simulink model "doublemass"  (R2018a)
settings: Solver=FixedStepAuto  StartTime=0.0  StopTime=10.0  FixedStep=0.02  RelTol=1e-3
values from neighbouring files (symbols this model uses):
  a_max = [10,]    [doublemass_para.m]
  a_min = [-10,]    [doublemass_para.m]
  adva_max = [0.001,0.001,0.001,0.001,]    [doublemass_para.m]
  adva_min = [-0.001,-0.001,-0.001,-0.001,]    [doublemass_para.m]
  ka = 50    [doublemass_para.m]
  m1 = 10    [doublemass_para.m]
  m2 = 10    [doublemass_para.m]
  x_ini = [x1_o, x1dot_o, x2_o, x2dot_o,]    [doublemass_para.m]
  x_max = [9999, 9999, 9999, 9999,]    [doublemass_para.m]
  x_min = [-9999, -9999, -9999, -9999,]    [doublemass_para.m]
libraries: simulink x1
settings Model: TunableVars=a_max,a_min,adva_max,adva_min,x_ini,x_max,x_min  TunableVarsStorageClass=Auto,Auto,Auto,Auto,Auto,Auto,Auto  TunableVarsTypeQualifier=,,,,,,  OrderedModelArguments=off  Creator=hjzsj  LastModifiedBy=Jet
settings DataIOCC: ReturnWorkspaceOutputs=on
settings OptimizationCC: DefaultParameterBehavior=Inlined  UseDivisionForNetSlopeComputation=on  UseFloatMulNetSlope=on  PassReuseOutputArgsAs=Individual arguments  NoFixptDivByZeroProtection=on  EfficientFloat2IntCast=on  LifeSpan=1  OptimizeBlockOrder=speed  DifferentSizesBufferReuse=on
settings DebuggingCC: ParameterTunabilityLossMsg=error
settings HardwareCC: ProdLongLongMode=on
settings SFSimCC: SimUseLocalCustomCode=on  MATLABDynamicMemAlloc=off
settings RTWCC: SystemTargetFile=ert.tlc  GenCodeOnly=on  TemplateMakefile=ert_default_tmf  PostCodeGenCommand=mat2json  RTWUseLocalCustomCode=on  TargetLang=C++
settings CodeAppCC: ForceParamTrailComments=on  IgnoreCustomStorageClasses=off  OperatorAnnotations=on  SimulinkDataObjDesc=on  SFDataObjDesc=on  CustomSymbolStrGlobalVar=rt$N$M  CustomSymbolStrType=$N$M  CustomSymbolStrFcn=$N$M$F  CustomSymbolStrMacro=$N$M  InsertBlockDesc=on
settings ERTTargetCC: TargetLangStandard=C++03 (ISO)  GenerateSampleERTMain=on  CombineSignalStateStructs=on  MultiInstanceERTCode=on  CodeInterfacePackaging=C++ class  SupportComplex=off  SupportContinuousTime=on  InlinedParameterPlacement=NonHierarchical  RootIOFormat=Structure reference  ERTCustomFileTemplate=example_file_process.tlc  ERTFilePackagingFormat=CompactWithDataFile

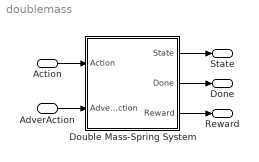
== system doublemass ==
  Action : Inport
  AdverAction : Inport  Port=2
  Double Mass-Spring System : Subsystem
  State : Outport  VectorParamsAs1DForOutWhenUnconnected=on
  Done : Outport  Port=2  VectorParamsAs1DForOutWhenUnconnected=on
  Reward : Outport  Port=3  VectorParamsAs1DForOutWhenUnconnected=on
  wires:
  Double Mass-Spring System/1(State) -> State/1
  Double Mass-Spring System/2(Done) -> Done/1
  Action/1 -> Double Mass-Spring System/1(Action)
  Double Mass-Spring System/3(Reward) -> Reward/1
  AdverAction/1 -> Double Mass-Spring System/2(AdverAction)

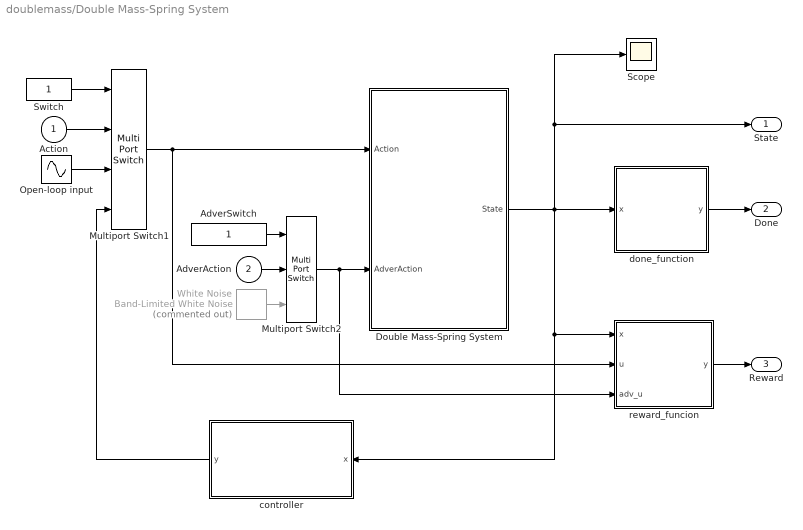
== system doublemass/Double Mass-Spring System ==
  Action : Inport
  AdverAction : Inport  Port=2
  AdverSwitch : Constant
  Double Mass-Spring System : Subsystem
  Multiport Switch1 : MultiPortSwitch
  Multiport Switch2 : MultiPortSwitch  Inputs=2
  Open-loop input : Sin  SampleTime=0
  Scope : Scope
  Switch : Constant
  White Noise : simulink/Sources/Band-Limited White Noise  Commented=on  Cov=[0.5]  Ts=0.02  seed=[23341]
  controller : MATLAB Function  TreatAsAtomicUnit=on
  done_function : MATLAB Function  TreatAsAtomicUnit=on
  reward_funcion : MATLAB Function  TreatAsAtomicUnit=on
  State : Outport  VectorParamsAs1DForOutWhenUnconnected=on
  Done : Outport  Port=2  VectorParamsAs1DForOutWhenUnconnected=on
  Reward : Outport  Port=3  VectorParamsAs1DForOutWhenUnconnected=on
  wires:
  done_function/1(y) -> Done/1
  reward_funcion/1(y) -> Reward/1
  controller/1(y) -> Multiport Switch1/4
  Switch/1 -> Multiport Switch1/1
  Action/1 -> Multiport Switch1/2
  Double Mass-Spring System/1(State) -> controller/1(x), reward_funcion/1(x), done_function/1(x), Scope/1, State/1
  Multiport Switch1/1 -> reward_funcion/2(u), Double Mass-Spring System/1(Action)
  Open-loop input/1 -> Multiport Switch1/3
  Multiport Switch2/1 -> reward_funcion/3(adv_u), Double Mass-Spring System/2(AdverAction)
  AdverSwitch/1 -> Multiport Switch2/1
  White Noise/1 -> Multiport Switch2/3
  AdverAction/1 -> Multiport Switch2/2

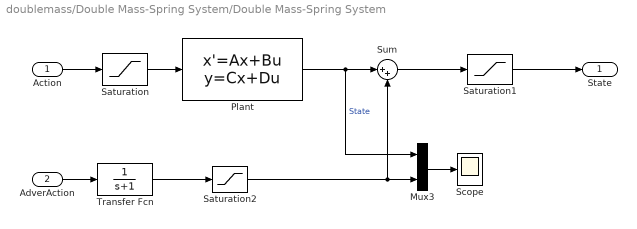
== system doublemass/Double Mass-Spring System/Double Mass-Spring System ==
  Action : Inport
  AdverAction : Inport  Port=2
  Mux3 : Mux  Inputs=2
  Plant : StateSpace  A=[0 1 0 0; -ka/m1 0 ka/m1 0; 0 0 0 1;ka/m2 0 -ka/m2 0]  B=[0; 1; 0; 0]  C=[1 0 0 0;0 1 0 0;0 0 1 0;0 0 0 1]  D=zeros(4,1)  InitialCondition=x_ini
  Saturation : Saturate  UpperLimit=a_max  LowerLimit=a_min
  Saturation1 : Saturate  UpperLimit=x_max  LowerLimit=x_min
  Saturation2 : Saturate  UpperLimit=adva_max  LowerLimit=adva_min
  Scope : Scope
  Sum : Sum  Inputs=|++
  Transfer Fcn : TransferFcn  Denominator=[1 1]
  State : Outport  VectorParamsAs1DForOutWhenUnconnected=on
  wires:
  Saturation/1 -> Plant/1
  Action/1 -> Saturation/1
  Saturation1/1 -> State/1
  Transfer Fcn/1 -> Saturation2/1
  Mux3/1 -> Scope/1
  AdverAction/1 -> Transfer Fcn/1
  Saturation2/1 -> Sum/2, Mux3/2
  Sum/1 -> Saturation1/1
  Plant/1 -> Mux3/1, Sum/1  "State"

== matlab function doublemass/Double Mass-Spring System/controller ==
  data: x input size=4; y output
function y = fcn(x)
done = (abs(x(1)) > 2.4)||(abs(x(3)) > 0.2094);
y = done;

== matlab function doublemass/Double Mass-Spring System/done_function ==
  data: x input; y output
function y = fcn(x)
done = (  (abs(x(3))>5) || ((abs(x(3)-0)<0.01) && (abs(x(4))<0.01)) || (x(3)>x(1))  );
y = done;

== matlab function doublemass/Double Mass-Spring System/reward_funcion ==
  data: x input; y output; u input; adv_u input
function y = fcn(x, u, adv_u)
reward = -(x(3)-0)^2-5*(x(4)-0)^2-0.2*u^2;
y = reward;
